simulink model "The_Entire_Control_Algorithm"  (R2024b)
settings: Solver=FixedStepDiscrete  StartTime=0.0  StopTime=10.0  FixedStep=0.001  RelTol=1e-3
undefined symbols (not defined in the file or in its folder): dspblkCoreblockFVToolHelper, gcbh
libraries: arduinolib x21, slpidlib x6, simulink x5, sharedTrackingLibrary x1
(part 2 of 2)

== matlab function The_Entire_Control_Algorithm/FEEDBACK LİNEARIZATION TERS KUVVETLİ ==
  data: d2q_des1 input; F output; d2q_des2 input; d2q_des3 input; states input
function F  = fcn(d2q_des1, d2q_des2, d2q_des3, states)

theta1 = states(1);
theta2 = states(2);
theta3 = states(3);
D_THETA_1 = states(4);
D_THETA_2 = states(5);
D_THETA_3 = states(6);


T1 =  -0.00018*D_THETA_1*D_THETA_2*sin(theta2) - 3.42e-5*D_THETA_1*D_THETA_2*sin(theta2 + theta3) - 3.078e-5*D_THETA_1*D_THETA_3*sin(theta3) - 3.42e-5*D_THETA_1*D_THETA_3*sin(theta2 + theta3) - 9.0e-5*(D_THETA_2^2)*sin(theta2) - 1.71e-5*(D_THETA_2^2)*sin(theta2 + theta3) - 3.078e-5*D_THETA_2*D_THETA_3*sin(theta3) - 3.42e-5*D_THETA_2*D_THETA_3*sin(theta2 + theta3) - 1.539e-5*(D_THETA_3^2)*sin(theta3) - 1.71e-5*(D_THETA_3^2)*sin(theta2 + theta3) + d2q_des1*(0.00018*cos(theta2) + 3.078e-5*cos(theta3) + 3.42e-5*cos(theta2 + theta3) + 0.000296104833333333) + d2q_des2*(9.0e-5*cos(theta2) + 3.078e-5*cos(theta3) + 1.71e-5*cos(theta2 + theta3) + 9.77715e-5) + d2q_des3*(1.539e-5*cos(theta3) + 1.71e-5*cos(theta2 + theta3) + 1.13715e-5) + 0.018639*cos(theta1) + 0.008829*cos(theta1 + theta2) + 0.00167751*cos(theta1 + theta2 + theta3) ;
T2 =  9.0e-5*(D_THETA_1^2)*sin(theta2) + 1.71e-5*(D_THETA_1^2)*sin(theta2 + theta3) - 3.078e-5*D_THETA_1*D_THETA_3*sin(theta3) - 3.078e-5*D_THETA_2*D_THETA_3*sin(theta3) - 1.539e-5*(D_THETA_3^2)*sin(theta3) + d2q_des1*(9.0e-5*cos(theta2) + 3.078e-5*cos(theta3) + 1.71e-5*cos(theta2 + theta3) + 9.77715e-5) + d2q_des2*(3.078e-5*cos(theta3) + 9.77715e-5) + d2q_des3*(1.539e-5*cos(theta3) + 1.13715e-5) + 0.008829*cos(theta1 + theta2) + 0.00167751*cos(theta1 + theta2 + theta3) ;
T3 =  1.539e-5*(D_THETA_1^2)*sin(theta3) + 1.71e-5*(D_THETA_1^2)*sin(theta2 + theta3) + 3.078e-5*D_THETA_1*D_THETA_2*sin(theta3) + 1.539e-5*(D_THETA_2^2)*sin(theta3) + d2q_des1*(1.539e-5*cos(theta3) + 1.71e-5*cos(theta2 + theta3) + 1.13715e-5) + d2q_des2*(1.539e-5*cos(theta3) + 1.13715e-5) + 1.13715e-5*d2q_des3 + 0.00167751*cos(theta1 + theta2 + theta3) ;


if T1<0
    F1 = T1/-0.005;
    F2 = -F1;
else
    F2 = T1/0.005;
    F1 = -F2;
end

if T2<0
    F3 = T2/-0.005;
    F4 = -F3;
else
    F4 = T2/0.005;
    F3 = -F4;
end

if T3<0
    F5 = T3/-0.005;
    F6 = -F5;
else
    F6 = T3/0.005;
    F5 = -F6;
end

F = [F1; F2; F3; F4; F5; F6];

end

== matlab function The_Entire_Control_Algorithm/EMPEDANS KONTROL2/MATLAB Function ==
  data: qe1 input; u1 output; dqe1 input; d2qe1 input; u2 output; u3 output; qe2 input; dqe2 input; d2qe2 input; qe3 input; dqe3 input; d2qe3 input
function [u1, u2, u3] = fcn(qe1, dqe1, d2qe1, qe2, dqe2, d2qe2, qe3, dqe3, d2qe3)

u1 = 0.001*d2qe1 + 7.5*dqe1 + 10*qe1 ;
u2 = 0.0009*d2qe2 + 6.75*dqe2 + 9*qe2 ;
u3 = 0.00057*d2qe3 + 4.275*dqe3 + 5.7*qe3 ;

end

== matlab function The_Entire_Control_Algorithm/MOTOR 1 KONTROL/MATLAB Function ==
  data: pwmRaw input; AIN1 output; AIN2 output
function [AIN1, AIN2] = fcn(pwmRaw)

if pwmRaw > 0
    AIN1=0;
    AIN2=1;
elseif pwmRaw <0 
    AIN1=1;
    AIN2=0;
else
    AIN1=0;
    AIN2=0;
end


end

== matlab function The_Entire_Control_Algorithm/MOTOR 2 KONTROL/MATLAB Function ==
  data: pwmRaw input; AIN1 output; AIN2 output
function [AIN1, AIN2] = fcn(pwmRaw)

if pwmRaw > 0
    AIN1=0;
    AIN2=1;
elseif pwmRaw <0 
    AIN1=1;
    AIN2=0;
else
    AIN1=0;
    AIN2=0;
end


end

== matlab function The_Entire_Control_Algorithm/MOTOR 3 KONTROL/MATLAB Function ==
  data: pwmRaw input; AIN1 output; AIN2 output
function [AIN1, AIN2] = fcn(pwmRaw)

if pwmRaw > 0
    AIN1=0;
    AIN2=1;
elseif pwmRaw <0 
    AIN1=1;
    AIN2=0;
else
    AIN1=0;
    AIN2=0;
end


end

== matlab function The_Entire_Control_Algorithm/MOTOR 4 KONTROL/MATLAB Function ==
  data: pwmRaw input; AIN1 output; AIN2 output
function [AIN1, AIN2] = fcn(pwmRaw)

if pwmRaw > 0
    AIN1=0;
    AIN2=1;
elseif pwmRaw <0 
    AIN1=1;
    AIN2=0;
else
    AIN1=0;
    AIN2=0;
end


end

== matlab function The_Entire_Control_Algorithm/MOTOR 5 KONTROL/MATLAB Function ==
  data: pwmRaw input; AIN1 output; AIN2 output
function [AIN1, AIN2] = fcn(pwmRaw)

if pwmRaw > 0
    AIN1=0;
    AIN2=1;
elseif pwmRaw <0 
    AIN1=1;
    AIN2=0;
else
    AIN1=0;
    AIN2=0;
end


end

== matlab function The_Entire_Control_Algorithm/MOTOR 6 KONTROL/MATLAB Function ==
  data: pwmRaw input; AIN1 output; AIN2 output
function [AIN1, AIN2] = fcn(pwmRaw)

if pwmRaw > 0
    AIN1=0;
    AIN2=1;
elseif pwmRaw <0 
    AIN1=1;
    AIN2=0;
else
    AIN1=0;
    AIN2=0;
end


end
